simulink model "check_jacob"  (R2018a)
settings: Solver=FixedStepAuto  StartTime=0.0  StopTime=6.14  FixedStep=ST  RelTol=1e-3
values from neighbouring files (symbols this model uses):
  delta = 0    [main.m]
  f = 610    [main.m]
  h = 0.05    [main.m]
  K = [f 0 0;0 f 0; 0 0 1]    [main.m]
  obj_points = [1.2 0.1 -0.2;1.2 -0.1 -0.2;1 0.1 -0.2;1 -0.1 -0.2]'    [main.m]
  x_ref = [0; 0; 0]    [main.m]
settings Model: Creator=hkedw  LastModifiedBy=hkedw

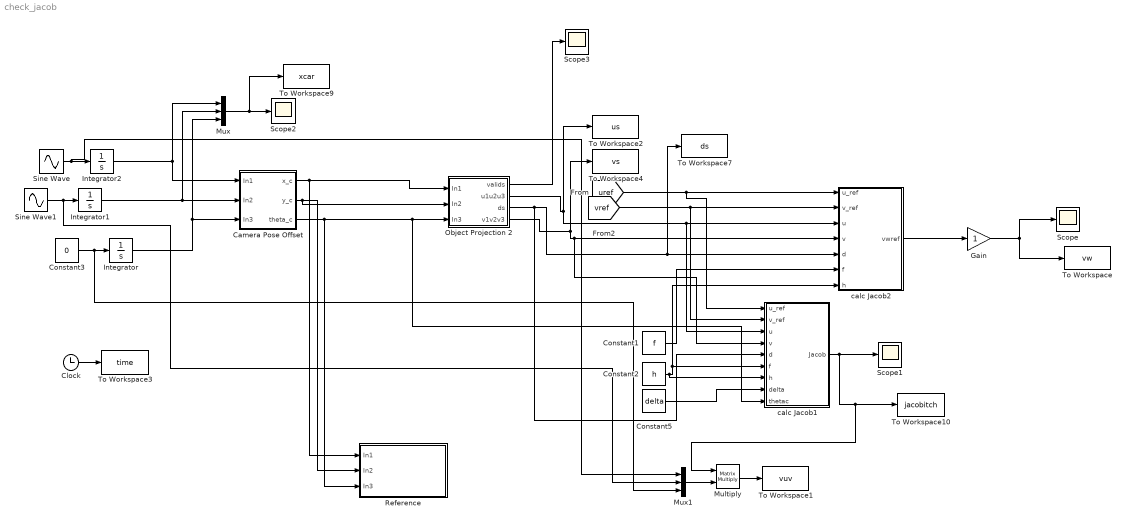
== system check_jacob ==
  Camera Pose Offset : Subsystem
  Clock : Clock
  Constant1 : Constant  Value=f
  Constant2 : Constant  Value=h
  Constant3 : Constant  Value=0
  Constant5 : Constant  Value=delta
  Gain : Gain
  Integrator : Integrator
  Integrator1 : Integrator
  Integrator2 : Integrator  InitialCondition=-1
  Multiply : Product  Multiplication=Matrix(*)
  Mux : Mux  Inputs=3
  Mux1 : Mux  Inputs=3
  Object Projection 2 : Subsystem
  Reference : Subsystem
  Scope{,1..3} (4 alike) : Scope
  Sine Wave : Sin  Amplitude=0.5  SampleTime=0
  Sine Wave1 : Sin  Amplitude=0.5  Phase=pi/2  SampleTime=0
  To Workspace : ToWorkspace  VariableName=vw  SaveFormat=Timeseries  SampleTime=-1
  To Workspace1 : ToWorkspace  VariableName=vuv  SaveFormat=Timeseries  SampleTime=-1
  To Workspace10 : ToWorkspace  VariableName=jacobitch  SaveFormat=Timeseries  SampleTime=-1
  To Workspace2 : ToWorkspace  VariableName=us  SaveFormat=Timeseries  SampleTime=-1
  To Workspace3 : ToWorkspace  VariableName=time  SaveFormat=Timeseries  SampleTime=-1
  To Workspace4 : ToWorkspace  VariableName=vs  SaveFormat=Timeseries  SampleTime=-1
  To Workspace7 : ToWorkspace  VariableName=ds  SaveFormat=Timeseries  SampleTime=-1
  To Workspace9 : ToWorkspace  VariableName=xcar  SaveFormat=Timeseries  SampleTime=-1
  calc Jacob1 : MATLAB Function  TreatAsAtomicUnit=on
  calc Jacob2 : MATLAB Function  TreatAsAtomicUnit=on
  wires:
  Integrator2/1 -> Camera Pose Offset/1(In1), Mux/1
  Integrator1/1 -> Mux/2, Camera Pose Offset/2(In2)
  Camera Pose Offset/2(y_c) -> Reference/2(In2), Object Projection 2/2(In2)
  Camera Pose Offset/3(theta_c) -> Reference/3(In3), Object Projection 2/3(In3), calc Jacob1/9(thetac)
  Object Projection 2/1(valids) -> Scope3/1
  Object Projection 2/2(u1u2u3) -> calc Jacob1/3(u), calc Jacob2/3(u), To Workspace2/1
  Constant1/1 -> calc Jacob2/6(f)
  Constant2/1 -> calc Jacob1/7(h), calc Jacob2/7(h), calc Jacob1/6(f)
  Gain/1 -> Scope/1, To Workspace/1
  calc Jacob2/1(vwref) -> Gain/1
  Mux/1 -> To Workspace9/1, Scope2/1
  Integrator/1 -> Mux/3, Camera Pose Offset/3(In3)
  Clock/1 -> To Workspace3/1
  Object Projection 2/4(v1v2v3) -> To Workspace4/1, calc Jacob1/4(v), calc Jacob2/4(v)
  [uref] -> calc Jacob1/1(u_ref), calc Jacob2/1(u_ref)
  [vref] -> calc Jacob1/2(v_ref), calc Jacob2/2(v_ref)
  Constant5/1 -> calc Jacob1/8(delta)
  Object Projection 2/3(ds) -> calc Jacob1/5(d), To Workspace7/1, calc Jacob2/5(d)
  calc Jacob1/1(Jacob) -> Multiply/1, To Workspace10/1, Scope1/1
  Camera Pose Offset/1(x_c) -> Reference/1(In1), Object Projection 2/1(In1)
  Mux1/1 -> Multiply/2
  Multiply/1 -> To Workspace1/1
  Constant3/1 -> Mux1/3, Integrator/1
  Sine Wave/1 -> Mux1/1, Integrator2/1
  Sine Wave1/1 -> Mux1/2, Integrator1/1

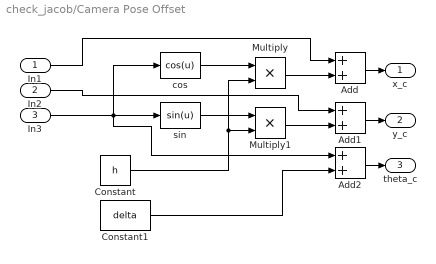
== system check_jacob/Camera Pose Offset ==
  In1 : Inport
  In2 : Inport  Port=2
  In3 : Inport  Port=3
  Add : Sum
  Add1 : Sum
  Add2 : Sum
  Constant : Constant  Value=h
  Constant1 : Constant  Value=delta
  Multiply : Product
  Multiply1 : Product
  cos : MATLABFcn  MATLABFcn=cos(u)
  sin : MATLABFcn  MATLABFcn=sin(u)
  x_c : Outport
  y_c : Outport  Port=2
  theta_c : Outport  Port=3
  wires:
  Multiply/1 -> Add/2
  cos/1 -> Multiply/1
  In1/1 -> Add/1
  In3/1 -> Add2/1, cos/1, sin/1
  sin/1 -> Multiply1/1
  Constant1/1 -> Add2/2
  Multiply1/1 -> Add1/2
  Constant/1 -> Multiply1/2, Multiply/2
  In2/1 -> Add1/1
  Add1/1 -> y_c/1
  Add2/1 -> theta_c/1
  Add/1 -> x_c/1

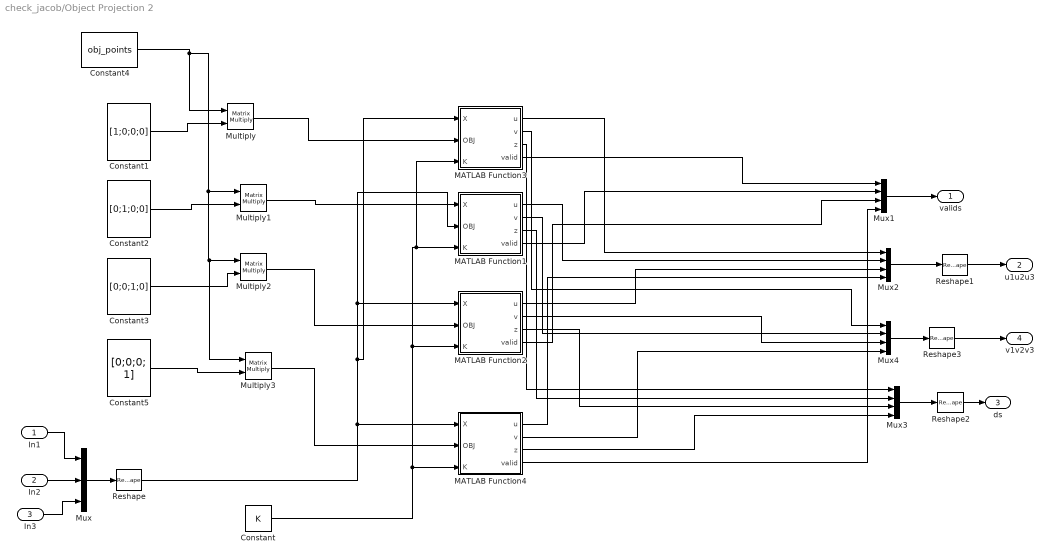
== system check_jacob/Object Projection 2 ==
  In1 : Inport
  In2 : Inport  Port=2
  In3 : Inport  Port=3
  Constant : Constant  Value=K  VectorParams1D=off
  Constant1 : Constant  Value=[1;0;0;0]  VectorParams1D=off
  Constant2 : Constant  Value=[0;1;0;0]  VectorParams1D=off
  Constant3 : Constant  Value=[0;0;1;0]  VectorParams1D=off
  Constant4 : Constant  Value=obj_points
  Constant5 : Constant  Value=[0;0;0; 1]  VectorParams1D=off
  MATLAB Function1 : MATLAB Function  TreatAsAtomicUnit=on
  MATLAB Function2 : MATLAB Function  TreatAsAtomicUnit=on
  MATLAB Function3 : MATLAB Function  TreatAsAtomicUnit=on
  MATLAB Function4 : MATLAB Function  TreatAsAtomicUnit=on
  Multiply{,1..3} (4 alike) : Product  Multiplication=Matrix(*)
  Mux : Mux  Inputs=3
  Mux{1..4} (4 alike) : Mux
  Reshape : Reshape  OutputDimensionality=Customize  OutputDimensions=[3,1]
  Reshape1 : Reshape  OutputDimensionality=Customize  OutputDimensions=[4,1]
  Reshape2 : Reshape  OutputDimensionality=Column vector (2-D)
  Reshape3 : Reshape  OutputDimensionality=Customize  OutputDimensions=[4,1]
  valids : Outport
  u1u2u3 : Outport  Port=2
  ds : Outport  Port=3
  v1v2v3 : Outport  Port=4
  wires:
  Constant3/1 -> Multiply2/2
  Constant2/1 -> Multiply1/2
  Constant4/1 -> Multiply/1, Multiply3/1, Multiply2/1, Multiply1/1
  Constant1/1 -> Multiply/2
  Mux1/1 -> valids/1
  In1/1 -> Mux/1
  In2/1 -> Mux/2
  Mux2/1 -> Reshape1/1
  Mux/1 -> Reshape/1
  Mux3/1 -> Reshape2/1
  Reshape1/1 -> u1u2u3/1
  Reshape2/1 -> ds/1
  In3/1 -> Mux/3
  Reshape/1 -> MATLAB Function2/1(X), MATLAB Function1/1(X), MATLAB Function3/1(X), MATLAB Function4/1(X)
  Multiply2/1 -> MATLAB Function2/2(OBJ)
  Multiply1/1 -> MATLAB Function1/2(OBJ)
  Constant/1 -> MATLAB Function3/3(K), MATLAB Function1/3(K), MATLAB Function2/3(K), MATLAB Function4/3(K)
  MATLAB Function3/1(u) -> Mux2/1
  MATLAB Function1/1(u) -> Mux2/2
  MATLAB Function1/2(v) -> Mux4/2
  MATLAB Function2/1(u) -> Mux2/3
  Mux4/1 -> Reshape3/1
  Reshape3/1 -> v1v2v3/1
  MATLAB Function3/2(v) -> Mux4/1
  MATLAB Function2/2(v) -> Mux4/3
  MATLAB Function2/3(z) -> Mux3/3
  MATLAB Function3/3(z) -> Mux3/1
  MATLAB Function1/3(z) -> Mux3/2
  MATLAB Function2/4(valid) -> Mux1/3
  MATLAB Function1/4(valid) -> Mux1/2
  MATLAB Function3/4(valid) -> Mux1/1
  Multiply/1 -> MATLAB Function3/2(OBJ)
  Constant5/1 -> Multiply3/2
  Multiply3/1 -> MATLAB Function4/2(OBJ)
  MATLAB Function4/4(valid) -> Mux1/4
  MATLAB Function4/3(z) -> Mux3/4
  MATLAB Function4/2(v) -> Mux4/4
  MATLAB Function4/1(u) -> Mux2/4

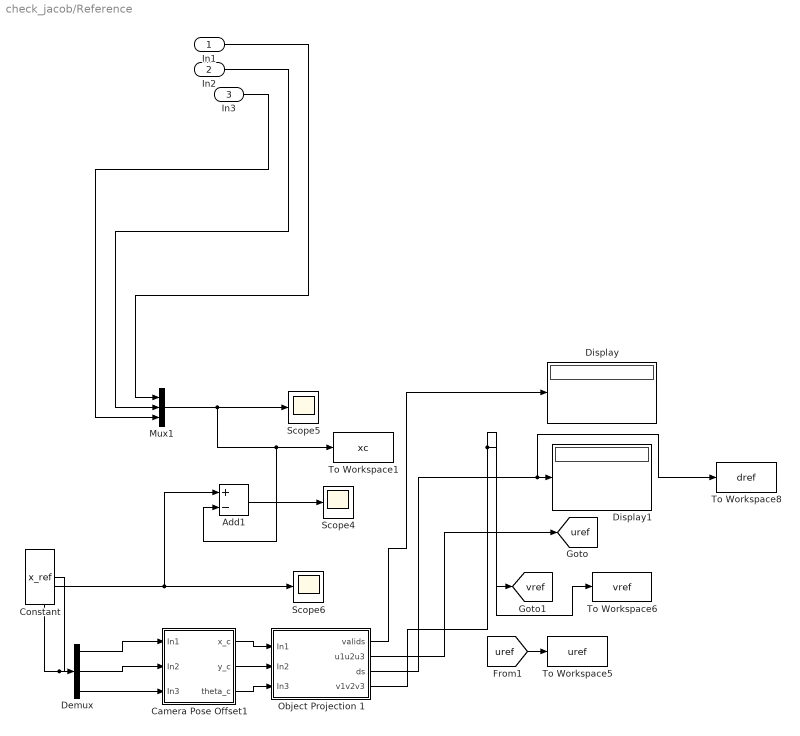
== system check_jacob/Reference ==
  In1 : Inport
  In2 : Inport  Port=2
  In3 : Inport  Port=3
  Add1 : Sum  Inputs=+-
  Camera Pose Offset1 : Subsystem
  Constant : Constant  Value=x_ref  VectorParams1D=off
  Demux : Demux  Outputs=3
  Display : Display
  Display1 : Display
  Mux1 : Mux  Inputs=3
  Object Projection 1 : Subsystem
  Scope4 : Scope
  Scope5 : Scope
  Scope6 : Scope
  To Workspace1 : ToWorkspace  VariableName=xc  SaveFormat=Timeseries  SampleTime=-1
  To Workspace5 : ToWorkspace  VariableName=uref  SaveFormat=Timeseries  SampleTime=-1
  To Workspace6 : ToWorkspace  VariableName=vref  SaveFormat=Timeseries  SampleTime=-1
  To Workspace8 : ToWorkspace  VariableName=dref  SaveFormat=Timeseries  SampleTime=-1
  tag scope: uref=global, vref=global
  wires:
  Mux1/1 -> To Workspace1/1, Add1/2, Scope5/1
  Add1/1 -> Scope4/1
  Constant/1 -> Add1/1, Scope6/1, Demux/1
  In2/1 -> Mux1/2
  Demux/1 -> Camera Pose Offset1/1(In1)
  Demux/2 -> Camera Pose Offset1/2(In2)
  Object Projection 1/1(valids) -> Display/1
  Camera Pose Offset1/2(y_c) -> Object Projection 1/2(In2)
  Object Projection 1/3(ds) -> To Workspace8/1, Display1/1
  Object Projection 1/4(v1v2v3) -> [vref], To Workspace6/1
  [uref] -> To Workspace5/1
  Object Projection 1/2(u1u2u3) -> [uref]
  Camera Pose Offset1/3(theta_c) -> Object Projection 1/3(In3)
  Demux/3 -> Camera Pose Offset1/3(In3)
  Camera Pose Offset1/1(x_c) -> Object Projection 1/1(In1)
  In3/1 -> Mux1/3
  In1/1 -> Mux1/1

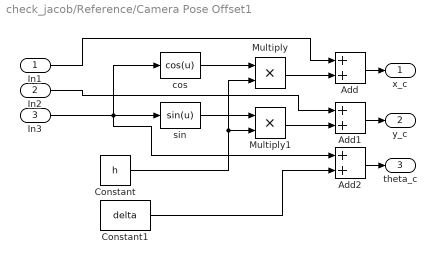
== system check_jacob/Reference/Camera Pose Offset1 ==
  In1 : Inport
  In2 : Inport  Port=2
  In3 : Inport  Port=3
  Add : Sum
  Add1 : Sum
  Add2 : Sum
  Constant : Constant  Value=h
  Constant1 : Constant  Value=delta
  Multiply : Product
  Multiply1 : Product
  cos : MATLABFcn  MATLABFcn=cos(u)
  sin : MATLABFcn  MATLABFcn=sin(u)
  x_c : Outport
  y_c : Outport  Port=2
  theta_c : Outport  Port=3
  wires:
  Multiply/1 -> Add/2
  cos/1 -> Multiply/1
  In1/1 -> Add/1
  In3/1 -> Add2/1, cos/1, sin/1
  sin/1 -> Multiply1/1
  Constant1/1 -> Add2/2
  Multiply1/1 -> Add1/2
  Constant/1 -> Multiply1/2, Multiply/2
  In2/1 -> Add1/1
  Add1/1 -> y_c/1
  Add2/1 -> theta_c/1
  Add/1 -> x_c/1

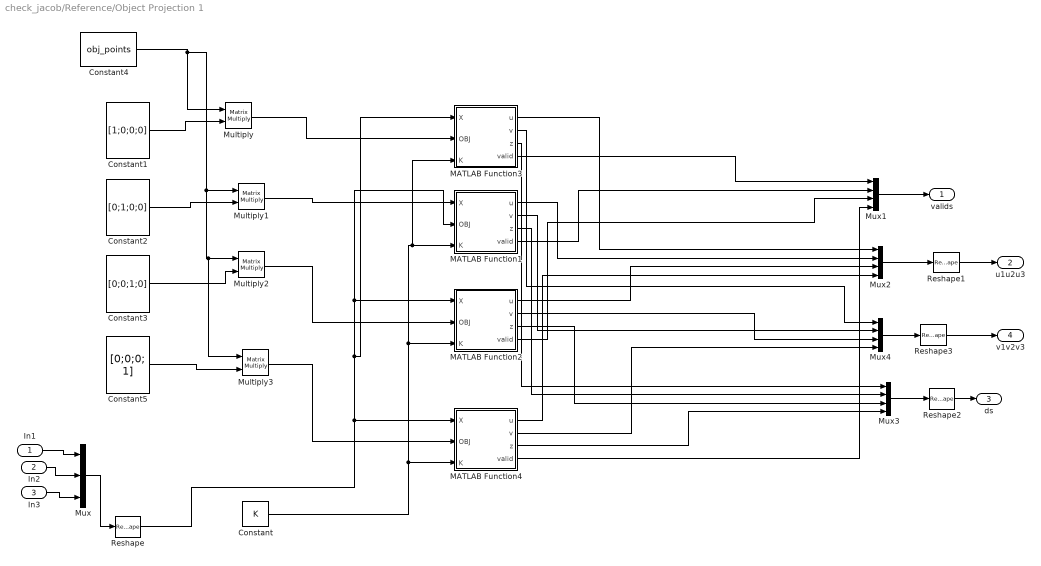
== system check_jacob/Reference/Object Projection 1 ==
  In1 : Inport
  In2 : Inport  Port=2
  In3 : Inport  Port=3
  Constant : Constant  Value=K  VectorParams1D=off
  Constant1 : Constant  Value=[1;0;0;0]  VectorParams1D=off
  Constant2 : Constant  Value=[0;1;0;0]  VectorParams1D=off
  Constant3 : Constant  Value=[0;0;1;0]  VectorParams1D=off
  Constant4 : Constant  Value=obj_points
  Constant5 : Constant  Value=[0;0;0; 1]  VectorParams1D=off
  MATLAB Function1 : MATLAB Function  TreatAsAtomicUnit=on
  MATLAB Function2 : MATLAB Function  TreatAsAtomicUnit=on
  MATLAB Function3 : MATLAB Function  TreatAsAtomicUnit=on
  MATLAB Function4 : MATLAB Function  TreatAsAtomicUnit=on
  Multiply{,1..3} (4 alike) : Product  Multiplication=Matrix(*)
  Mux : Mux  Inputs=3
  Mux{1..4} (4 alike) : Mux
  Reshape : Reshape  OutputDimensionality=Customize  OutputDimensions=[3,1]
  Reshape1 : Reshape  OutputDimensionality=Customize  OutputDimensions=[4,1]
  Reshape2 : Reshape  OutputDimensionality=Column vector (2-D)
  Reshape3 : Reshape  OutputDimensionality=Customize  OutputDimensions=[4,1]
  valids : Outport
  u1u2u3 : Outport  Port=2
  ds : Outport  Port=3
  v1v2v3 : Outport  Port=4
  wires:
  Constant3/1 -> Multiply2/2
  Constant2/1 -> Multiply1/2
  Constant4/1 -> Multiply/1, Multiply3/1, Multiply2/1, Multiply1/1
  Constant1/1 -> Multiply/2
  Mux1/1 -> valids/1
  In1/1 -> Mux/1
  In2/1 -> Mux/2
  Mux2/1 -> Reshape1/1
  Mux/1 -> Reshape/1
  Mux3/1 -> Reshape2/1
  Reshape1/1 -> u1u2u3/1
  Reshape2/1 -> ds/1
  In3/1 -> Mux/3
  Reshape/1 -> MATLAB Function2/1(X), MATLAB Function1/1(X), MATLAB Function3/1(X), MATLAB Function4/1(X)
  Multiply2/1 -> MATLAB Function2/2(OBJ)
  Multiply1/1 -> MATLAB Function1/2(OBJ)
  Constant/1 -> MATLAB Function3/3(K), MATLAB Function1/3(K), MATLAB Function2/3(K), MATLAB Function4/3(K)
  MATLAB Function3/1(u) -> Mux2/1
  MATLAB Function1/1(u) -> Mux2/2
  MATLAB Function1/2(v) -> Mux4/2
  MATLAB Function2/1(u) -> Mux2/3
  Mux4/1 -> Reshape3/1
  Reshape3/1 -> v1v2v3/1
  MATLAB Function3/2(v) -> Mux4/1
  MATLAB Function2/2(v) -> Mux4/3
  MATLAB Function2/3(z) -> Mux3/3
  MATLAB Function3/3(z) -> Mux3/1
  MATLAB Function1/3(z) -> Mux3/2
  MATLAB Function2/4(valid) -> Mux1/3
  MATLAB Function1/4(valid) -> Mux1/2
  MATLAB Function3/4(valid) -> Mux1/1
  Multiply/1 -> MATLAB Function3/2(OBJ)
  Constant5/1 -> Multiply3/2
  Multiply3/1 -> MATLAB Function4/2(OBJ)
  MATLAB Function4/4(valid) -> Mux1/4
  MATLAB Function4/3(z) -> Mux3/4
  MATLAB Function4/2(v) -> Mux4/4
  MATLAB Function4/1(u) -> Mux2/4

== matlab function check_jacob/Reference/Object Projection 1/MATLAB Function1 ==
  data: X input; u output; OBJ input; K input; v output; z output; valid output
function [u,v,z,valid]=projection(X,OBJ,K)
%%%%%%%
% X = [xc,yc,thetac] 
% OBJ = [xo,yo,zo]
%%%%%%
% assert size(X,1) == 3
% assert size(X,2) == 1
% assert size(K,1) == 3
% assert size(K,2) == 3
% assert size(OBJ,1) == 3
% assert size(OBJ,2) == 1

%%%%%
% conversion
% todo
%%%%%



%%%%%
% Rotate to camera 
%%%%%
Cta = X(3);
Rinv = [cos(Cta),sin(Cta);-sin(Cta),cos(Cta)];
X_c = Rinv*(OBJ(1:2,1)-X(1:2,1));
x_c = -X_c(2);
y_c=OBJ(3);
z_c = X_c(1);

if z_c == 0
    u = 0;
    v = 0;
    z = 0;
    valid = 0;
    return;
end
imagepoints=K*[x_c/z_c;y_c/z_c;1];

u = imagepoints(1);
v = imagepoints(2);
z = z_c;
valid = 1;


end

== matlab function check_jacob/Reference/Object Projection 1/MATLAB Function2 ==
  data: X input; u output; OBJ input; K input; v output; z output; valid output
function [u,v,z,valid]=projection(X,OBJ,K)
%%%%%%%
% X = [xc,yc,thetac] 
% OBJ = [xo,yo,zo]
%%%%%%
% assert size(X,1) == 3
% assert size(X,2) == 1
% assert size(K,1) == 3
% assert size(K,2) == 3
% assert size(OBJ,1) == 3
% assert size(OBJ,2) == 1

%%%%%
% conversion
% todo
%%%%%



%%%%%
% Rotate to camera 
%%%%%
Cta = X(3);
Rinv = [cos(Cta),sin(Cta);-sin(Cta),cos(Cta)];
X_c = Rinv*(OBJ(1:2,1)-X(1:2,1));
x_c = -X_c(2);
y_c=OBJ(3);
z_c = X_c(1);

if z_c == 0
    u = 0;
    v = 0;
    z = 0;
    valid = 0;
    return;
end
imagepoints=K*[x_c/z_c;y_c/z_c;1];

u = imagepoints(1);
v = imagepoints(2);
z = z_c;
valid = 1;


end

== matlab function check_jacob/calc Jacob2 ==
  data: u_ref input; v_ref input; u input; v input; vwref output; d input; f input; h input
function vwref  = fcn(u_ref,v_ref,u,v,d,f,h)
uref = reshape(u_ref,4,1);
vref = reshape(v_ref,4,1);


u = reshape(u,4,1);
v = reshape(v,4,1);
d = reshape(d,4,1);

uJacob = [u./d 1./d*h*f-f-u.*u/f];
vJacob = [v./d u.*v/f];

% vwref = pinv(uJacob)*(uref-u);
vwref = pinv([uJacob;vJacob])*[uref-u;vref-v];
% vwref = pinv(vJacob)*(vref-v);

== matlab function check_jacob/Object Projection 2/MATLAB Function1 ==
  data: X input; u output; OBJ input; K input; v output; z output; valid output
function [u,v,z,valid]=projection(X,OBJ,K)
%%%%%%%
% X = [xc,yc,thetac] 
% OBJ = [xo,yo,zo]
%%%%%%
% assert size(X,1) == 3
% assert size(X,2) == 1
% assert size(K,1) == 3
% assert size(K,2) == 3
% assert size(OBJ,1) == 3
% assert size(OBJ,2) == 1

%%%%%
% conversion
% todo
%%%%%



%%%%%
% Rotate to camera 
%%%%%
Cta = X(3);
Rinv = [cos(Cta),sin(Cta);-sin(Cta),cos(Cta)];
X_c = Rinv*(OBJ(1:2,1)-X(1:2,1));
x_c = -X_c(2);
y_c=OBJ(3);
z_c = X_c(1);

if z_c == 0
    u = 0;
    v = 0;
    z = 0;
    valid = 0;
    return;
end
imagepoints=K*[x_c/z_c;y_c/z_c;1];

u = imagepoints(1);
v = imagepoints(2);
z = z_c;
valid = 1;


end

== matlab function check_jacob/Object Projection 2/MATLAB Function2 ==
  data: X input; u output; OBJ input; K input; v output; z output; valid output
function [u,v,z,valid]=projection(X,OBJ,K)
%%%%%%%
% X = [xc,yc,thetac] 
% OBJ = [xo,yo,zo]
%%%%%%
% assert size(X,1) == 3
% assert size(X,2) == 1
% assert size(K,1) == 3
% assert size(K,2) == 3
% assert size(OBJ,1) == 3
% assert size(OBJ,2) == 1

%%%%%
% conversion
% todo
%%%%%



%%%%%
% Rotate to camera 
%%%%%
Cta = X(3);
Rinv = [cos(Cta),sin(Cta);-sin(Cta),cos(Cta)];
X_c = Rinv*(OBJ(1:2,1)-X(1:2,1));
x_c = -X_c(2);
y_c=OBJ(3);
z_c = X_c(1);

if z_c == 0
    u = 0;
    v = 0;
    z = 0;
    valid = 0;
    return;
end
imagepoints=K*[x_c/z_c;y_c/z_c;1];

u = imagepoints(1);
v = imagepoints(2);
z = z_c;
valid = 1;


end

== matlab function check_jacob/Object Projection 2/MATLAB Function3 ==
  data: X input; u output; OBJ input; K input; v output; z output; valid output
function [u,v,z,valid]=projection(X,OBJ,K)
%%%%%%%
% X = [xc,yc,thetac] 
% OBJ = [xo,yo,zo]
%%%%%%
% assert size(X,1) == 3
% assert size(X,2) == 1
% assert size(K,1) == 3
% assert size(K,2) == 3
% assert size(OBJ,1) == 3
% assert size(OBJ,2) == 1

%%%%%
% conversion
% todo
%%%%%



%%%%%
% Rotate to camera 
%%%%%
Cta = X(3);
Rinv = [cos(Cta),sin(Cta);-sin(Cta),cos(Cta)];
X_c = Rinv*(OBJ(1:2,1)-X(1:2,1));
x_c = -X_c(2);
y_c=OBJ(3);
z_c = X_c(1);

if z_c == 0
    u = 0;
    v = 0;
    z = 0;
    valid = 0;
    return;
end
imagepoints=K*[x_c/z_c;y_c/z_c;1];

u = imagepoints(1);
v = imagepoints(2);
z = z_c;
valid = 1;


end

== matlab function check_jacob/Reference/Object Projection 1/MATLAB Function3 ==
  data: X input; u output; OBJ input; K input; v output; z output; valid output
function [u,v,z,valid]=projection(X,OBJ,K)
%%%%%%%
% X = [xc,yc,thetac] 
% OBJ = [xo,yo,zo]
%%%%%%
% assert size(X,1) == 3
% assert size(X,2) == 1
% assert size(K,1) == 3
% assert size(K,2) == 3
% assert size(OBJ,1) == 3
% assert size(OBJ,2) == 1

%%%%%
% conversion
% todo
%%%%%



%%%%%
% Rotate to camera 
%%%%%
Cta = X(3);
Rinv = [cos(Cta),sin(Cta);-sin(Cta),cos(Cta)];
X_c = Rinv*(OBJ(1:2,1)-X(1:2,1));
x_c = -X_c(2);
y_c=OBJ(3);
z_c = X_c(1);

if z_c == 0
    u = 0;
    v = 0;
    z = 0;
    valid = 0;
    return;
end
imagepoints=K*[x_c/z_c;y_c/z_c;1];

u = imagepoints(1);
v = imagepoints(2);
z = z_c;
valid = 1;


end

== matlab function check_jacob/Object Projection 2/MATLAB Function4 ==
  data: X input; u output; OBJ input; K input; v output; z output; valid output
function [u,v,z,valid]=projection(X,OBJ,K)
%%%%%%%
% X = [xc,yc,thetac] 
% OBJ = [xo,yo,zo]
%%%%%%
% assert size(X,1) == 3
% assert size(X,2) == 1
% assert size(K,1) == 3
% assert size(K,2) == 3
% assert size(OBJ,1) == 3
% assert size(OBJ,2) == 1

%%%%%
% conversion
% todo
%%%%%



%%%%%
% Rotate to camera 
%%%%%
Cta = X(3);
Rinv = [cos(Cta),sin(Cta);-sin(Cta),cos(Cta)];
X_c = Rinv*(OBJ(1:2,1)-X(1:2,1));
x_c = -X_c(2);
y_c=OBJ(3);
z_c = X_c(1);

if z_c == 0
    u = 0;
    v = 0;
    z = 0;
    valid = 0;
    return;
end
imagepoints=K*[x_c/z_c;y_c/z_c;1];

u = imagepoints(1);
v = imagepoints(2);
z = z_c;
valid = 1;


end

== matlab function check_jacob/Reference/Object Projection 1/MATLAB Function4 ==
  data: X input; u output; OBJ input; K input; v output; z output; valid output
function [u,v,z,valid]=projection(X,OBJ,K)
%%%%%%%
% X = [xc,yc,thetac] 
% OBJ = [xo,yo,zo]
%%%%%%
% assert size(X,1) == 3
% assert size(X,2) == 1
% assert size(K,1) == 3
% assert size(K,2) == 3
% assert size(OBJ,1) == 3
% assert size(OBJ,2) == 1

%%%%%
% conversion
% todo
%%%%%



%%%%%
% Rotate to camera 
%%%%%
Cta = X(3);
Rinv = [cos(Cta),sin(Cta);-sin(Cta),cos(Cta)];
X_c = Rinv*(OBJ(1:2,1)-X(1:2,1));
x_c = -X_c(2);
y_c=OBJ(3);
z_c = X_c(1);

if z_c == 0
    u = 0;
    v = 0;
    z = 0;
    valid = 0;
    return;
end
imagepoints=K*[x_c/z_c;y_c/z_c;1];

u = imagepoints(1);
v = imagepoints(2);
z = z_c;
valid = 1;


end

== matlab function check_jacob/calc Jacob1 ==
  data: u_ref input; v_ref input; u input; v input; Jacob output; d input; f input; h input; delta input; thetac input
function Jacob  = fcn(u_ref,v_ref,u,v,d,f,h,delta,thetac)

uref = reshape(u_ref,4,1);
vref = reshape(v_ref,4,1);


u = reshape(u,4,1);
v = reshape(v,4,1);
d = reshape(d,4,1);

uJacob = [-f*sin(thetac)./d+u./d*cos(thetac), f*cos(thetac)./d+u./d*sin(thetac), h*f./d+f*+u.*u/f];% something is wrong?
vJacob = [v./d*cos(thetac) v./d*sin(thetac) v./d*h*sin(delta)+u.*v/f];% this part is ok

Jacob = [uJacob;vJacob];
% xycref = pinv(uJacob)*(uref-u);
% xycref = pinv([uJacob;vJacob])*[uref-u;vref-v];
%  xycref = pinv(vJacob)*(vref-v);
